simulink subsystem "AdasCorePlantModel"  (R2023a)
settings: Solver=VariableStepAuto  StartTime=0.0  StopTime=10.0  RelTol=1e-3
undefined symbols (not defined in the file or in its folder): BalNotActWait, BalOffWait, BalOnWait, Battery, contactorTime, CtrlBcuTrlrBrkGain, CtrlTcuInitGear, CtrlVcuCltch1InitCmd, CtrlVcuEvChrgLmtBpt, CtrlVcuEvRegenBrkCutOff, CtrlVcuEvRegenBrkSpdBpt, CtrlVcuEvSocBpt, currentFactor, CV_Gain, DiscIntNeverNeededParam, EnvAbsPrs, EnvAirTemp, EnvNomFrictionScaling, EnvNominalGrade, EnvWindVelX, EnvWindVelY, EnvWindVelZ, flgEnBalancing, HighTempLimit, I_cc, LowTempLimit, MaxCellVoltThrsld, MaxChrgCurrLim, MaxDchrgCurrLim, MinCellVoltDchrgCurrentLim_BP, MinCellVoltDchrgCurrentLim_Table, noCurrent, OverCellVoltageLimit, PlntBattModNumCellPar, PlntBattModNumCellSer, PlntBattNumMod, PlntBattSocInit, PlntBattTempInitDegC, PlntBrkActrBoreFrnt, PlntBrkFrntBias, PlntBrkKinFricCffFrnt, PlntBrkNumPadsFrnt, PlntBrkPadMeanRadiusFrnt, PlntBrkPrsFctr, PlntBrkRearBias, PlntDiffrntlRatio, PlntEM1EffTbl, PlntEM1Spd, PlntEM1Trq, PlntEM1TrqEff, PlntVehDstCGFrntAxl, PlntVehDstCGRearAxl, SnsrFltThld, TargetDeltaV, timeoutContactor, timeoutCurrent, Ts, UnderCellVoltageLimit, voltThreshold, vRatio
libraries: simulink x10, sharedTrackingLibrary x2, autolibutils x1
(part 1 of 4)
settings Model: Creator=sam  LastModifiedBy=sam

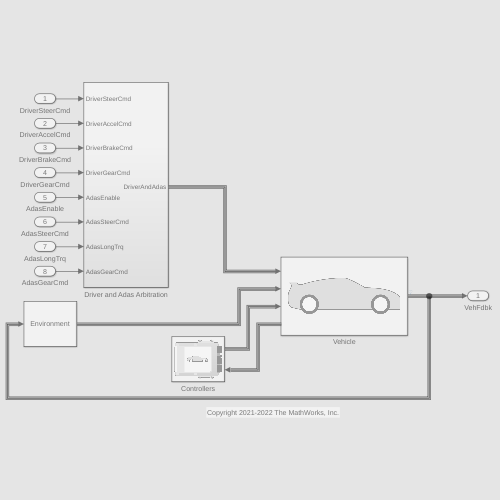
[thumbnail: Simulink's stored preview of the top-level diagram]
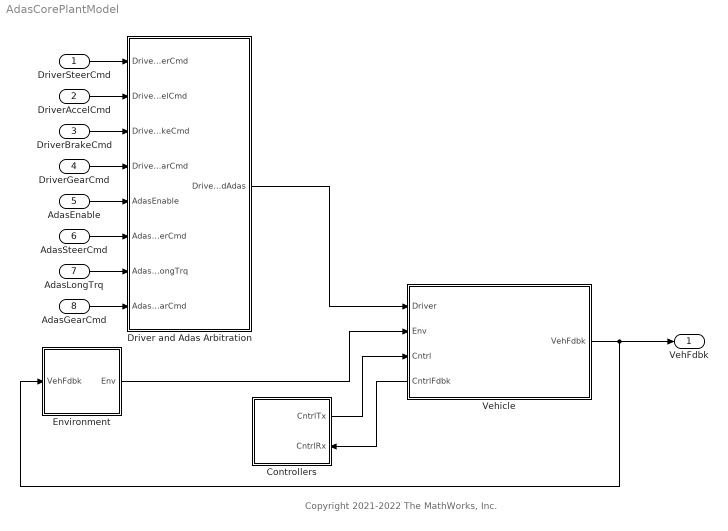
== system AdasCorePlantModel ==
  note: Copyright 2021-2022 The MathWorks, Inc.
  DriverSteerCmd : Inport
  DriverAccelCmd : Inport  Port=2
  DriverBrakeCmd : Inport  Port=3
  DriverGearCmd : Inport  Port=4
  AdasEnable : Inport  Port=5
  AdasSteerCmd : Inport  Port=6
  AdasLongTrq : Inport  Port=7
  AdasGearCmd : Inport  Port=8
  Controllers : Subsystem
      settings: PortSchema="{\"entries\":[{\"content\":{\"sides\":[{\"content\":{\"connectorIds\":[]},\"type\":\"ConnectorPlacement.EquallySpacedRectSide\",\"uuid\":\"a925dd9c-6905-4c67-a62c-b22bb69d2bd6\"},{\"content\":{\"connectorIds\":[\"Out1\",\"In1\"],\"side\":\"RIGHT\"},\"type\":\"ConnectorPlacement.EquallySpacedRectSide\",\"uuid\":\"9930ed3e-43a4-46d4-b9ee-7ed64fae32ef\"},{\"content\":{\"connectorIds\":[],\"side\":\"TOP\"},\"type\":\"ConnectorPlacement.EquallySpacedRectSide\",\"uuid\":\"68d2ac4e-de3d-40d3-8b44-059f2a72a6bc\"}]},\"type\":\"ConnectorPlacement.EquallySpacedConnector\",\"uuid\":\"c0be7d07-475b-4046-8bfa-76004f6da9b2\"}],\"packageUris\":[\"http://schema.mathworks.com/mf0/Connector/R2020b\"],\"version\":\"1.0\"}"
      mask Display: image('SystemControllers.png')
  Driver and Adas Arbitration : Subsystem
  Environment : Subsystem
      mask Display: disp('Environment')
  Vehicle : Subsystem
      settings: PortSchema="{\"entries\":[{\"content\":{\"sides\":[{\"content\":{\"connectorIds\":[\"In1\",\"In2\",\"In3\",\"Out2\"]},\"type\":\"ConnectorPlacement.EquallySpacedRectSide\",\"uuid\":\"5a3b6452-81f2-4c00-bf1f-ccfcf792e289\"},{\"content\":{\"connectorIds\":[\"Out1\"],\"side\":\"RIGHT\"},\"type\":\"ConnectorPlacement.EquallySpacedRectSide\",\"uuid\":\"1578d241-3f7e-42c3-aed7-11454fa326bd\"},{\"content\":{\"connectorIds\":[],\"side\":\"TOP\"},\"type\":\"ConnectorPlacement.EquallySpacedRectSide\",\"uuid\":\"4d307cdf-4623-4beb-9171-96c6b8eb862e\"}]},\"type\":\"ConnectorPlacement.EquallySpacedConnector\",\"uuid\":\"daa9e8ca-739b-480d-9fe9-9a76305e5c3d\"}],\"packageUris\":[\"http://schema.mathworks.com/mf0/Connector/R2020b\"],\"version\":\"1.0\"}"
      mask Display: image('PassengerVehicle.png')
  VehFdbk : Outport
  wires:
  Environment/1(Env) -> Vehicle/2(Env)
  DriverSteerCmd/1 -> Driver and Adas Arbitration/1(DriverSteerCmd)
  DriverAccelCmd/1 -> Driver and Adas Arbitration/2(DriverAccelCmd)
  Vehicle/1(VehFdbk) -> VehFdbk/1, Environment/1(VehFdbk)
  AdasGearCmd/1 -> Driver and Adas Arbitration/8(AdasGearCmd)
  Controllers/1(CntrlTx) -> Vehicle/3(Cntrl)
  DriverGearCmd/1 -> Driver and Adas Arbitration/4(DriverGearCmd)
  AdasLongTrq/1 -> Driver and Adas Arbitration/7(AdasLongTrq)
  AdasEnable/1 -> Driver and Adas Arbitration/5(AdasEnable)
  AdasSteerCmd/1 -> Driver and Adas Arbitration/6(AdasSteerCmd)
  Driver and Adas Arbitration/1(DriverAndAdas) -> Vehicle/1(Driver)
  DriverBrakeCmd/1 -> Driver and Adas Arbitration/3(DriverBrakeCmd)
  Vehicle/2(CntrlFdbk) -> Controllers/1(CntrlRx)

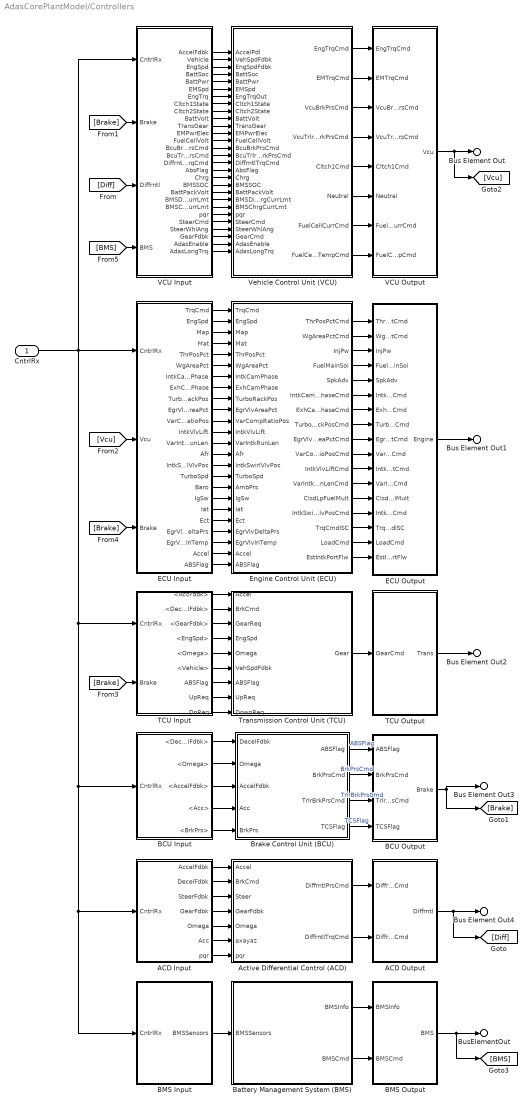
== system AdasCorePlantModel/Controllers ==
  CntrlRx : Inport
  ACD Input : Subsystem
  ACD Output : Subsystem
  Active Differential Control (ACD) : Subsystem  Variant=on  VariantControlMode=label  LabelModeActiveChoice=Choice
  BCU Input : Subsystem
  BCU Output : Subsystem
  BMS Input : Subsystem
  BMS Output : Subsystem
  Battery Management System (BMS) : Subsystem  Variant=on  VariantControlMode=label  LabelModeActiveChoice=Choice
  Brake Control Unit (BCU) : Subsystem  Variant=on  VariantControlMode=label  LabelModeActiveChoice=Choice
  ECU Input : Subsystem
  ECU Output : Subsystem
  Engine Control Unit (ECU) : Subsystem  Variant=on  VariantControlMode=label  LabelModeActiveChoice=No Engine Controller
  TCU Input : Subsystem
  TCU Output : Subsystem
  Transmission Control Unit (TCU) : Subsystem  Variant=on  VariantControlMode=label  VariantControl=Variant1  LabelModeActiveChoice=Choice
  VCU Input : Subsystem
  VCU Output : Subsystem
  Vehicle Control Unit (VCU) : Subsystem  Variant=on  VariantControlMode=label  LabelModeActiveChoice=Choice
  Bus Element Out : Outport  PortName=CntrlTx  Element=Vcu
  Bus Element Out1 : Outport  PortName=CntrlTx  Element=Engine
  Bus Element Out2 : Outport  PortName=CntrlTx  Element=Trans
  Bus Element Out3 : Outport  PortName=CntrlTx  Element=Brake
  Bus Element Out4 : Outport  PortName=CntrlTx  Element=Diff
  BusElementOut : Outport  PortName=CntrlTx  Element=BMS
  wires:
  ECU Input/1(TrqCmd) -> Engine Control Unit (ECU)/1(TrqCmd)
  CntrlRx/1 -> VCU Input/1(CntrlRx), ECU Input/1(CntrlRx), BMS Input/1(CntrlRx), ACD Input/1(CntrlRx), BCU Input/1(CntrlRx), TCU Input/1(CntrlRx)
  VCU Input/1(AccelFdbk) -> Vehicle Control Unit (VCU)/1(AccelPdl)
  VCU Input/2(Vehicle) -> Vehicle Control Unit (VCU)/2(VehSpdFdbk)
  VCU Input/3(EngSpd) -> Vehicle Control Unit (VCU)/3(EngSpdFdbk)
  VCU Input/4(BattSoc) -> Vehicle Control Unit (VCU)/4(BattSoc)
  VCU Input/5(BattPwr) -> Vehicle Control Unit (VCU)/5(BattPwr)
  VCU Input/6(EMSpd) -> Vehicle Control Unit (VCU)/6(EMSpd)
  VCU Input/7(EngTrq) -> Vehicle Control Unit (VCU)/7(EngTrqOut)
  VCU Input/8(Cltch1State) -> Vehicle Control Unit (VCU)/8(Cltch1State)
  VCU Input/9(Cltch2State) -> Vehicle Control Unit (VCU)/9(Cltch2State)
  VCU Input/10(BattVolt) -> Vehicle Control Unit (VCU)/10(BattVolt)
  VCU Input/11(TransGear) -> Vehicle Control Unit (VCU)/11(TransGear)
  VCU Input/12(EMPwrElec) -> Vehicle Control Unit (VCU)/12(EMPwrElec)
  VCU Input/13(FuelCellVolt) -> Vehicle Control Unit (VCU)/13(FuelCellVolt)
  VCU Input/18(Chrg) -> Vehicle Control Unit (VCU)/18(Chrg)
  VCU Input/17(AbsFlag) -> Vehicle Control Unit (VCU)/17(AbsFlag)
  VCU Input/16(DiffrntlTrqCmd) -> Vehicle Control Unit (VCU)/16(DiffrntlTrqCmd)
  VCU Input/14(BcuBrkPrsCmd) -> Vehicle Control Unit (VCU)/14(BcuBrkPrsCmd)
  ECU Input/2(EngSpd) -> Engine Control Unit (ECU)/2(EngSpd)
  ECU Input/3(Map) -> Engine Control Unit (ECU)/3(Map)
  ECU Input/4(Mat) -> Engine Control Unit (ECU)/4(Mat)
  ECU Input/5(ThrPosPct) -> Engine Control Unit (ECU)/5(ThrPosPct)
  ECU Input/6(WgAreaPct) -> Engine Control Unit (ECU)/6(WgAreaPct)
  ECU Input/7(IntkCamPhase) -> Engine Control Unit (ECU)/7(IntkCamPhase)
  ECU Input/8(ExhCamPhase) -> Engine Control Unit (ECU)/8(ExhCamPhase)
  ECU Input/9(TurboRackPos) -> Engine Control Unit (ECU)/9(TurboRackPos)
  ECU Input/10(EgrVlvAreaPct) -> Engine Control Unit (ECU)/10(EgrVlvAreaPct)
  ECU Input/11(VarCompRatioPos) -> Engine Control Unit (ECU)/11(VarCompRatioPos)
  ECU Input/12(IntkVlvLift) -> Engine Control Unit (ECU)/12(IntkVlvLift)
  ECU Input/13(VarIntkRunLen) -> Engine Control Unit (ECU)/13(VarIntkRunLen)
  ECU Input/14(Afr) -> Engine Control Unit (ECU)/14(Afr)
  ECU Input/15(IntkSwirlVlvPos) -> Engine Control Unit (ECU)/15(IntkSwirlVlvPos)
  ECU Input/16(TurboSpd) -> Engine Control Unit (ECU)/16(TurboSpd)
  ECU Input/17(Baro) -> Engine Control Unit (ECU)/17(AmbPrs)
  ECU Input/18(IgSw) -> Engine Control Unit (ECU)/18(IgSw)
  ECU Input/19(Iat) -> Engine Control Unit (ECU)/19(Iat)
  ECU Input/20(Ect) -> Engine Control Unit (ECU)/20(Ect)
  ECU Input/21(EgrVlvDeltaPrs) -> Engine Control Unit (ECU)/21(EgrVlvDeltaPrs)
  ECU Input/22(EgrVlvInTemp) -> Engine Control Unit (ECU)/22(EgrVlvInTemp)
  TCU Input/8(UpReq) -> Transmission Control Unit (TCU)/8(UpReq)
  TCU Input/1(<AccFdbk>) -> Transmission Control Unit (TCU)/1(Accel)
  TCU Input/2(<DecelFdbk>) -> Transmission Control Unit (TCU)/2(BrkCmd)
  TCU Input/3(<GearFdbk>) -> Transmission Control Unit (TCU)/3(GearReq)
  TCU Input/4(<EngSpd>) -> Transmission Control Unit (TCU)/4(EngSpd)
  TCU Input/5(<Omega>) -> Transmission Control Unit (TCU)/5(Omega)
  TCU Input/6(<Vehicle>) -> Transmission Control Unit (TCU)/6(VehSpdFdbk)
  TCU Input/7(ABSFlag) -> Transmission Control Unit (TCU)/7(ABSFlag)
  TCU Input/9(DnReq) -> Transmission Control Unit (TCU)/9(DownReq)
  ACD Input/1(AccelFdbk) -> Active Differential Control (ACD)/1(Accel)
  ACD Input/2(DecelFdbk) -> Active Differential Control (ACD)/2(BrkCmd)
  ACD Input/3(SteerFdbk) -> Active Differential Control (ACD)/3(Steer)
  ACD Input/4(GearFdbk) -> Active Differential Control (ACD)/4(GearFdbk)
  ACD Input/5(Omega) -> Active Differential Control (ACD)/5(Omega)
  ACD Input/6(Acc) -> Active Differential Control (ACD)/6(axayaz)
  ACD Input/7(pqr) -> Active Differential Control (ACD)/7(pqr)
  Active Differential Control (ACD)/1(DiffrntlPrsCmd) -> ACD Output/1(DiffrntlPrsCmd)
  Active Differential Control (ACD)/2(DiffrntlTrqCmd) -> ACD Output/2(DiffrntlTrqCmd)
  ACD Output/1(Diffrntl) -> [Diff], Bus Element Out4/1
  Transmission Control Unit (TCU)/1(" Gear") -> TCU Output/1(GearCmd)
  TCU Output/1(Trans) -> Bus Element Out2/1
  Vehicle Control Unit (VCU)/1(EngTrqCmd) -> VCU Output/1(EngTrqCmd)
  Vehicle Control Unit (VCU)/2(EMTrqCmd) -> VCU Output/2(EMTrqCmd)
  Vehicle Control Unit (VCU)/3(VcuBrkPrsCmd) -> VCU Output/3(VcuBrkPrsCmd)
  Vehicle Control Unit (VCU)/5(Cltch1Cmd) -> VCU Output/5(Cltch1Cmd)
  Vehicle Control Unit (VCU)/6(Neutral) -> VCU Output/6(Neutral)
  Vehicle Control Unit (VCU)/7(FuelCellCurrCmd) -> VCU Output/7(FuelCellCurrCmd)
  Vehicle Control Unit (VCU)/8(FuelCellTempCmd) -> VCU Output/8(FuelCellTempCmd)
  BCU Output/1(Brake) -> Bus Element Out3/1, [Brake]
  Engine Control Unit (ECU)/1(ThrPosPctCmd) -> ECU Output/1(ThrPosPctCmd)
  Engine Control Unit (ECU)/2(WgAreaPctCmd) -> ECU Output/2(WgAreaPctCmd)
  Engine Control Unit (ECU)/3(InjPw) -> ECU Output/3(InjPw)
  Engine Control Unit (ECU)/4(FuelMainSoi) -> ECU Output/4(FuelMainSoi)
  Engine Control Unit (ECU)/5(SpkAdv) -> ECU Output/5(SpkAdv)
  Engine Control Unit (ECU)/6(IntkCamPhaseCmd) -> ECU Output/6(IntkCamPhaseCmd)
  Engine Control Unit (ECU)/7(ExhCamPhaseCmd) -> ECU Output/7(ExhCamPhaseCmd)
  Engine Control Unit (ECU)/8(TurboRackPosCmd) -> ECU Output/8(TurboRackPosCmd)
  Engine Control Unit (ECU)/9(EgrVlvAreaPctCmd) -> ECU Output/9(EgrVlvAreaPctCmd)
  Engine Control Unit (ECU)/10(VarCompRatioPosCmd) -> ECU Output/10(VarCompRatioPosCmd)
  Engine Control Unit (ECU)/11(IntkVlvLiftCmd) -> ECU Output/11(IntkVlvLiftCmd)
  Engine Control Unit (ECU)/12(VarIntkRunLenCmd) -> ECU Output/12(VarIntkRunLenCmd)
  Engine Control Unit (ECU)/13(ClsdLpFuelMult) -> ECU Output/13(ClsdLpFuelMult)
  Engine Control Unit (ECU)/14(IntkSwirlVlvPosCmd) -> ECU Output/14(IntkSwirlVlvPosCmd)
  Engine Control Unit (ECU)/15(TrqCmdISC) -> ECU Output/15(TrqCmdISC)
  Engine Control Unit (ECU)/16(LoadCmd) -> ECU Output/16(LoadCmd)
  Engine Control Unit (ECU)/17(EstIntkPortFlw) -> ECU Output/17(EstIntkPortFlw)
  VCU Output/1(Vcu) -> Bus Element Out/1, [Vcu]
  ECU Output/1(Engine) -> Bus Element Out1/1
  [Brake] -> VCU Input/2(Brake)
  [Diff] -> VCU Input/3(Diffrntl)
  [Vcu] -> ECU Input/2(Vcu)
  [Brake] -> TCU Input/2(Brake)
  ECU Input/23(Accel) -> Engine Control Unit (ECU)/23(Accel)
  ECU Input/24(ABSFlag) -> Engine Control Unit (ECU)/24(ABSFlag)
  [Brake] -> ECU Input/3(Brake)
  Brake Control Unit (BCU)/1(ABSFlag) -> BCU Output/1(ABSFlag)  "ABSFlag"
  Brake Control Unit (BCU)/2(BrkPrsCmd) -> BCU Output/2(BrkPrsCmd)  "BrkPrsCmd"
  Brake Control Unit (BCU)/4(TCSFlag) -> BCU Output/4(TCSFlag)  "TCSFlag"
  BCU Input/1(<DecelFdbk>) -> Brake Control Unit (BCU)/1(DecelFdbk)
  BCU Input/2(<Omega>) -> Brake Control Unit (BCU)/2(Omega)
  BCU Input/5(<BrkPrs>) -> Brake Control Unit (BCU)/5(BrkPrs)
  BCU Input/4(<Acc>) -> Brake Control Unit (BCU)/4(Acc)
  BCU Input/3(<AccelFdbk>) -> Brake Control Unit (BCU)/3(AccelFdbk)
  BMS Input/1(BMSSensors) -> Battery Management System (BMS)/1(BMSSensors)
  Battery Management System (BMS)/1(BMSInfo) -> BMS Output/1(BMSInfo)
  Battery Management System (BMS)/2(BMSCmd) -> BMS Output/2(BMSCmd)
  BMS Output/1(BMS) -> [BMS], BusElementOut/1
  [BMS] -> VCU Input/4(BMS)
  VCU Input/19(BMSSOC) -> Vehicle Control Unit (VCU)/19(BMSSOC)
  VCU Input/20(BattPackVolt) -> Vehicle Control Unit (VCU)/20(BattPackVolt)
  VCU Input/21(BMSDischrgCurrLmt) -> Vehicle Control Unit (VCU)/21(BMSDischrgCurrLmt)
  VCU Input/22(BMSChrgCurrLmt) -> Vehicle Control Unit (VCU)/22(BMSChrgCurrLmt)
  Brake Control Unit (BCU)/3(TrlrBrkPrsCmd) -> BCU Output/3(TrlrBrkPrsCmd)  "TrlrBrkPrsCmd"
  Vehicle Control Unit (VCU)/4(VcuTrlrBrkPrsCmd) -> VCU Output/4(VcuTrlrBrkPrsCmd)
  VCU Input/15(BcuTrlrBrkPrsCmd) -> Vehicle Control Unit (VCU)/15(BcuTrlrBrkPrsCmd)
  VCU Input/23(pqr) -> Vehicle Control Unit (VCU)/23(pqr)
  VCU Input/24(SteerCmd) -> Vehicle Control Unit (VCU)/24(SteerCmd)
  VCU Input/25(SteerWhlAng) -> Vehicle Control Unit (VCU)/25(SteerWhlAng)
  VCU Input/26(GearFdbk) -> Vehicle Control Unit (VCU)/26(GearCmd)
  VCU Input/27(AdasEnable) -> Vehicle Control Unit (VCU)/27(AdasEnable)
  VCU Input/28(AdasLongTrq) -> Vehicle Control Unit (VCU)/28(AdasLongTrq)

== system AdasCorePlantModel/Driver and Adas Arbitration ==
  DriverSteerCmd : Inport
  DriverAccelCmd : Inport  Port=2
  DriverBrakeCmd : Inport  Port=3
  DriverGearCmd : Inport  Port=4
  AdasEnable : Inport  Port=5
  AdasSteerCmd : Inport  Port=6
  AdasLongTrq : Inport  Port=7
  AdasGearCmd : Inport  Port=8
  Bus Creator : BusCreator  Inputs=5
  Constant : Constant
  Switch : Switch  Criteria=u2 > Threshold  SaturateOnIntegerOverflow=off  InputSameDT=off
  Switch1 : Switch  Criteria=u2 > Threshold  SaturateOnIntegerOverflow=off  InputSameDT=off
  DriverAndAdas : Outport
  tag scope: AdasEnable=global, AdasGearReq=global, AdasLongTorque=global, AdasSteerCmd=global, DriverAccelPedal=global, DriverBrakePedal=global, DriverGearReq=global, DriverSteerCmd=global
  wires:
  Bus Creator/1 -> DriverAndAdas/1
  Switch1/1 -> Bus Creator/1  "SteerCmd"
  [DriverAccelPedal] -> Bus Creator/2  "AccelCmd"
  [DriverBrakePedal] -> Bus Creator/3  "DecelCmd"
  Switch/1 -> Bus Creator/4  "GearCmd"
  Constant/1 -> Bus Creator/5  "IgnSwtch"
  [AdasGearReq] -> Switch/1
  [DriverGearReq] -> Switch/3  "GearCmd"
  [AdasEnable] -> Switch/2
  [DriverSteerCmd] -> Switch1/3
  [AdasSteerCmd] -> Switch1/1
  [AdasEnable] -> Switch1/2
  DriverSteerCmd/1 -> [DriverSteerCmd]
  DriverAccelCmd/1 -> [DriverAccelPedal]
  DriverBrakeCmd/1 -> [DriverBrakePedal]
  DriverGearCmd/1 -> [DriverGearReq]
  AdasEnable/1 -> [AdasEnable]
  AdasLongTrq/1 -> [AdasLongTorque]
  AdasSteerCmd/1 -> [AdasSteerCmd]
  AdasGearCmd/1 -> [AdasGearReq]

== system AdasCorePlantModel/Environment ==
  note: The Ground Feedback variant subsystem is automatically enabled/disabled according to the 3D Engine settings found in the Reference Generator.
      | Manually overriding this variant may result in initialization errors.
  In Bus Element8 : Inport  PortName=VehFdbk  Element=Body.InertFrm
  In Bus Element9 : Inport  PortName=VehFdbk  Element=Body.InertFrm
  In Bus Element1 : Inport  PortName=VehFdbk  Element=Body.InertFrm.Cg.Disp
  BusElementIn3 : Inport  PortName=VehFdbk  Element=Wheels.Wheels.z
  BusElementIn1 : Inport  PortName=VehFdbk  Element=Wheels.Wheels.Omega
  BusElementIn : Inport  PortName=VehFdbk  Element=Suspension.SuspChassis.Whl.Ang
  Baro_Pa : Constant  Value=EnvAbsPrs  SampleTime=0
  Bus Creator : BusCreator  Inputs=3
  Bus Creator1 : BusCreator  Inputs=5
  Constant3 : Constant  Value=EnvWindVelX  SampleTime=0
  Constant4 : Constant  Value=EnvWindVelY  SampleTime=0
  Constant5 : Constant  Value=EnvWindVelZ  SampleTime=0
  Estimated Grade : Subsystem
  Ground Feedback : Subsystem  Variant=on  VariantControlMode=label  LabelModeActiveChoice=0
  Temp_degK : Constant  Value=EnvAirTemp  SampleTime=0
  Varying Friction : Subsystem  Variant=on  VariantControlMode=label  VariantControl=Choice  LabelModeActiveChoice=0
  Vector Concatenate : Concatenate  NumInputs=3
  Env : Outport  VectorParamsAs1DForOutWhenUnconnected=off
  wires:
  Constant5/1 -> Vector Concatenate/3  "Z"
  Vector Concatenate/1 -> Bus Creator1/3  "Wind"
  Constant3/1 -> Vector Concatenate/1  "X"
  Constant4/1 -> Vector Concatenate/2  "Y"
  Ground Feedback/1(Ground) -> Bus Creator1/5, Estimated Grade/1(Gnd)  "Gnd"
  Bus Creator1/1 -> Env/1
  Temp_degK/1 -> Bus Creator1/1  "Temp"
  Baro_Pa/1 -> Bus Creator1/2  "Baro"
  In Bus Element8/1 -> Varying Friction/1(In1)
  In Bus Element9/1 -> Varying Friction/2(In2)
  In Bus Element1/1 -> Varying Friction/3(Cg)
  Varying Friction/1(FricCoeffLambda) -> Ground Feedback/1(Friction)
  Estimated Grade/1(Grade) -> Bus Creator1/4  "Grade"
  BusElementIn3/1 -> Bus Creator/1  "z"
  BusElementIn1/1 -> Bus Creator/2  "Omega"
  BusElementIn/1 -> Bus Creator/3  "WhlAng"
  Bus Creator/1 -> Ground Feedback/2(WheelFdbk)  "WheelFdbk"

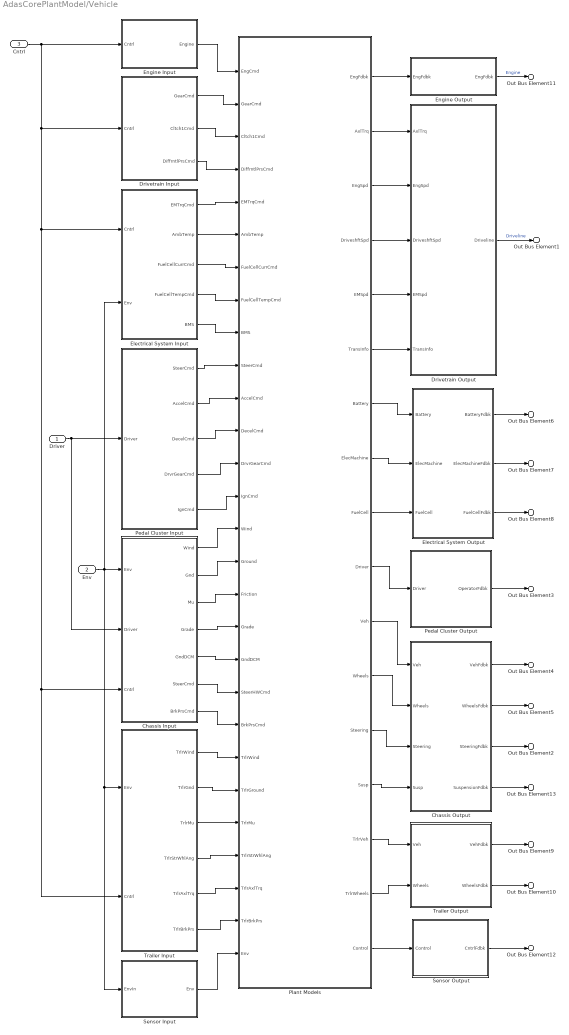
== system AdasCorePlantModel/Vehicle ==
  Driver : Inport
  Env : Inport  Port=2
  Cntrl : Inport  Port=3
  Chassis Input : Subsystem
  Chassis Output : Subsystem
  Drivetrain Input : Subsystem
  Drivetrain Output : Subsystem
  Electrical System Input : Subsystem
  Electrical System Output : Subsystem
  Engine Input : Subsystem
  Engine Output : Subsystem
  Pedal Cluster Input : Subsystem
  Pedal Cluster Output : Subsystem
  Plant Models : Subsystem  Variant=on  VariantControlMode=label  VariantControl=Choice  LabelModeActiveChoice=SimulinkModels
  Sensor Input : Subsystem
  Sensor Output : Subsystem
  Trailer Input : Subsystem
  Trailer Output : Subsystem
  Out Bus Element3 : Outport  PortName=VehFdbk  Element=Driver
  Out Bus Element4 : Outport  PortName=VehFdbk  Element=Body
  Out Bus Element5 : Outport  PortName=VehFdbk  Element=Wheels
  Out Bus Element1 : Outport  PortName=VehFdbk  Element=Driveline
  Out Bus Element2 : Outport  PortName=VehFdbk  Element=Steering
  Out Bus Element6 : Outport  PortName=VehFdbk  Element=Battery
  Out Bus Element7 : Outport  PortName=VehFdbk  Element=EM
  Out Bus Element8 : Outport  PortName=VehFdbk  Element=FuelCell
  Out Bus Element9 : Outport  PortName=VehFdbk  Element=TrlrBody
  Out Bus Element10 : Outport  PortName=VehFdbk  Element=TrlrWheels
  Out Bus Element11 : Outport  PortName=VehFdbk  Element=Engine
  Out Bus Element13 : Outport  PortName=VehFdbk  Element=Suspension
  Out Bus Element12 : Outport  Port=2  PortName=CntrlFdbk
  wires:
  Env/1 -> Electrical System Input/2(Env), Chassis Input/1(Env), Sensor Input/1(EnvIn), Trailer Input/1(Env)
  Driver/1 -> Chassis Input/2(Driver), Pedal Cluster Input/1(Driver)
  Pedal Cluster Output/1(OperatorFdbk) -> Out Bus Element3/1
  Chassis Output/2(WheelsFdbk) -> Out Bus Element5/1
  Chassis Output/1(VehFdbk) -> Out Bus Element4/1
  Drivetrain Output/1(Driveline) -> Out Bus Element1/1  "Driveline"
  Cntrl/1 -> Chassis Input/3(Cntrl), Trailer Input/2(Cntrl), Electrical System Input/1(Cntrl), Drivetrain Input/1(Cntrl), Engine Input/1(Cntrl)
  Chassis Output/3(SteeringFdbk) -> Out Bus Element2/1
  Electrical System Output/2(ElecMachineFdbk) -> Out Bus Element7/1
  Electrical System Output/1(BatteryFdbk) -> Out Bus Element6/1
  Electrical System Output/3(FuelCellFdbk) -> Out Bus Element8/1
  Trailer Output/2(WheelsFdbk) -> Out Bus Element10/1
  Trailer Output/1(VehFdbk) -> Out Bus Element9/1
  Engine Output/1(EngFdbk) -> Out Bus Element11/1  "Engine"
  Engine Input/1(Engine) -> Plant Models/1(EngCmd)
  Drivetrain Input/1(GearCmd) -> Plant Models/2(GearCmd)
  Drivetrain Input/2(Cltch1Cmd) -> Plant Models/3(Cltch1Cmd)
  Drivetrain Input/3(DiffrntlPrsCmd) -> Plant Models/4(DiffrntlPrsCmd)
  Electrical System Input/1(EMTrqCmd) -> Plant Models/5(EMTrqCmd)
  Electrical System Input/2(AmbTemp) -> Plant Models/6(AmbTemp)
  Electrical System Input/3(FuelCellCurrCmd) -> Plant Models/7(FuelCellCurrCmd)
  Electrical System Input/4(FuelCellTempCmd) -> Plant Models/8(FuelCellTempCmd)
  Pedal Cluster Input/1(SteerCmd) -> Plant Models/10(SteerCmd)
  Pedal Cluster Input/2(AccelCmd) -> Plant Models/11(AccelCmd)
  Pedal Cluster Input/3(DecelCmd) -> Plant Models/12(DecelCmd)
  Pedal Cluster Input/4(DrvrGearCmd) -> Plant Models/13(DrvrGearCmd)
  Pedal Cluster Input/5(IgnCmd) -> Plant Models/14(IgnCmd)
  Chassis Input/1(Wind) -> Plant Models/15(Wind)
  Chassis Input/2(Gnd) -> Plant Models/16(Ground)
  Chassis Input/3(Mu) -> Plant Models/17(Friction)
  Chassis Input/6(SteerCmd) -> Plant Models/20(SteerHWCmd)
  Chassis Input/7(BrkPrsCmd) -> Plant Models/21(BrkPrsCmd)
  Trailer Input/1(TrlrWind) -> Plant Models/22(TrlrWind)
  Trailer Input/2(TrlrGnd) -> Plant Models/23(TrlrGround)
  Trailer Input/3(TrlrMu) -> Plant Models/24(TrlrMu)
  Trailer Input/4(TrlrStrWhlAng) -> Plant Models/25(TrlrStrWhlAng)
  Trailer Input/5(TrlrAxlTrq) -> Plant Models/26(TrlrAxlTrq)
  Trailer Input/6(TrlrBrkPrs) -> Plant Models/27(TrlrBrkPrs)
  Plant Models/1(EngFdbk) -> Engine Output/1("EngFdbk ")
  Plant Models/2(AxlTrq) -> Drivetrain Output/1(AxlTrq)
  Plant Models/3(EngSpd) -> Drivetrain Output/2(EngSpd)
  Plant Models/4(DriveshftSpd) -> Drivetrain Output/3(DriveshftSpd)
  Plant Models/5(EMSpd) -> Drivetrain Output/4(EMSpd)
  Plant Models/6(TransInfo) -> Drivetrain Output/5(TransInfo)
  Plant Models/7(Battery) -> Electrical System Output/1(Battery)
  Plant Models/8(ElecMachine) -> Electrical System Output/2(ElecMachine)
  Plant Models/9(FuelCell) -> Electrical System Output/3(FuelCell)
  Plant Models/10(Driver) -> Pedal Cluster Output/1(Driver)
  Plant Models/11(Veh) -> Chassis Output/1(Veh)
  Plant Models/12(Wheels) -> Chassis Output/2(Wheels)
  Plant Models/13(Steering) -> Chassis Output/3(Steering)
  Plant Models/15(TrlrVeh) -> Trailer Output/1(Veh)
  Plant Models/16(TrlrWheels) -> Trailer Output/2(Wheels)
  Plant Models/17(Control) -> Sensor Output/1(Control)
  Sensor Output/1(CntrlFdbk) -> Out Bus Element12/1
  Sensor Input/1(Env) -> Plant Models/28(Env)
  Plant Models/14(Susp) -> Chassis Output/4(Susp)
  Chassis Output/4(SuspensionFdbk) -> Out Bus Element13/1
  Chassis Input/4(Grade) -> Plant Models/18(Grade)
  Electrical System Input/5(BMS) -> Plant Models/9(BMS)
  Chassis Input/5(GndDCM) -> Plant Models/19(GndDCM)

== system AdasCorePlantModel/Controllers/ACD Input ==
  CntrlRx : Inport
  Bus Selector3 : BusSelector  OutputSignals=Driver.AccelFdbk,Driver.DecelFdbk,Driver.SteerFdbk,Driver.GearFdbk,Wheels.Omega,IMU.Acc,IMU.pqr
  Rate Transition{1..7} (7 alike) : RateTransition  Deterministic=off
  AccelFdbk : Outport
  DecelFdbk : Outport  Port=2
  SteerFdbk : Outport  Port=3
  GearFdbk : Outport  Port=4
  Omega : Outport  Port=5
  Acc : Outport  Port=6
  pqr : Outport  Port=7
  wires:
  Bus Selector3/7 -> Rate Transition7/1  "<pqr>"
  Bus Selector3/3 -> Rate Transition2/1  "<SteerFdbk>"
  Bus Selector3/1 -> Rate Transition5/1  "<AccelFdbk>"
  Bus Selector3/6 -> Rate Transition6/1  "<Acc>"
  Bus Selector3/2 -> Rate Transition1/1  "<DecelFdbk>"
  Bus Selector3/4 -> Rate Transition3/1  "<GearFdbk>"
  Bus Selector3/5 -> Rate Transition4/1  "<Omega>"
  CntrlRx/1 -> Bus Selector3/1
  Rate Transition5/1 -> AccelFdbk/1
  Rate Transition1/1 -> DecelFdbk/1
  Rate Transition2/1 -> SteerFdbk/1
  Rate Transition3/1 -> GearFdbk/1
  Rate Transition4/1 -> Omega/1
  Rate Transition6/1 -> Acc/1
  Rate Transition7/1 -> pqr/1

== system AdasCorePlantModel/Controllers/ACD Output ==
  DiffrntlPrsCmd : Inport
  DiffrntlTrqCmd : Inport  Port=2
  Bus Creator4 : BusCreator  Inputs=2
  Diffrntl : Outport
  wires:
  DiffrntlPrsCmd/1 -> Bus Creator4/1  "DiffrntlPrsCmd"
  Bus Creator4/1 -> Diffrntl/1  "Diffrntl"
  DiffrntlTrqCmd/1 -> Bus Creator4/2  "DiffrntlTrqCmd"

== system AdasCorePlantModel/Controllers/Active Differential Control (ACD) ==
  note: 1) Add Subsystem or Model blocks as valid variant choices.
      | 2) You cannot connect blocks at this level. At simulation, connectivity is automatically
      | determined, based on the active variant and port name matching.
  Accel : Inport  PortDimensions=1
  BrkCmd : Inport  Port=2  PortDimensions=1
  Steer : Inport  Port=3
  GearFdbk : Inport  Port=4
  Omega : Inport  Port=5  Unit=rad/s  PortDimensions=4
  axayaz : Inport  Port=6
  pqr : Inport  Port=7
  No Control : Subsystem  VariantControl=No Control
  No Control (non-reference) : Subsystem  VariantControl=Choice
  DiffrntlPrsCmd : Outport  VectorParamsAs1DForOutWhenUnconnected=off
  DiffrntlTrqCmd : Outport  Port=2  VectorParamsAs1DForOutWhenUnconnected=off

== system AdasCorePlantModel/Controllers/BCU Input ==
  CntrlRx : Inport
  Bus Selector : BusSelector  OutputSignals=Driver.DecelFdbk,Wheels.Omega,Vehicle.xddot,Driver.AccelFdbk,Wheels.BrkPrs
  Rate Transition{1..5} (5 alike) : RateTransition  Deterministic=off
  <DecelFdbk> : Outport
  <Omega> : Outport  Port=2
  <AccelFdbk> : Outport  Port=3
  <Acc> : Outport  Port=4
  <BrkPrs> : Outport  Port=5
  wires:
  Bus Selector/4 -> Rate Transition3/1  "<AccelFdbk>"
  Bus Selector/5 -> Rate Transition4/1  "<BrkPrs>"
  Bus Selector/2 -> Rate Transition1/1  "<Omega>"
  CntrlRx/1 -> Bus Selector/1
  Bus Selector/1 -> Rate Transition5/1  "<DecelFdbk>"
  Bus Selector/3 -> Rate Transition2/1  "<xddot>"
  Rate Transition5/1 -> <DecelFdbk>/1
  Rate Transition1/1 -> <Omega>/1
  Rate Transition2/1 -> <Acc>/1
  Rate Transition3/1 -> <AccelFdbk>/1
  Rate Transition4/1 -> <BrkPrs>/1

== system AdasCorePlantModel/Controllers/BCU Output ==
  ABSFlag : Inport
  BrkPrsCmd : Inport  Port=2
  TrlrBrkPrsCmd : Inport  Port=3
  TCSFlag : Inport  Port=4
  Bus Creator2 : BusCreator  Inputs=4
  Brake : Outport
  wires:
  Bus Creator2/1 -> Brake/1  "Brake"
  BrkPrsCmd/1 -> Bus Creator2/2
  TCSFlag/1 -> Bus Creator2/4
  ABSFlag/1 -> Bus Creator2/1
  TrlrBrkPrsCmd/1 -> Bus Creator2/3

== system AdasCorePlantModel/Controllers/BMS Input ==
  CntrlRx : Inport
  Bus Selector3 : BusSelector  OutputSignals=Battery.BMSSensors
  BMSSensors : Outport
  wires:
  CntrlRx/1 -> Bus Selector3/1
  Bus Selector3/1 -> BMSSensors/1  "<BMSSensors>"

== system AdasCorePlantModel/Controllers/BMS Output ==
  BMSInfo : Inport
  BMSCmd : Inport  Port=2
  Bus Creator4 : BusCreator  Inputs=2
  BMS : Outport
  wires:
  BMSCmd/1 -> Bus Creator4/2  "BMSCmd"
  Bus Creator4/1 -> BMS/1  "BMS"
  BMSInfo/1 -> Bus Creator4/1  "BMSInfo"

== system AdasCorePlantModel/Controllers/Battery Management System (BMS) ==
  BMSSensors : Inport
  BMS (non-reference) : Subsystem  VariantControl=Choice
  Battery Management System : ModelReference  ModelNameDialog=BMSController.slx  SimulationMode=Normal  VariantControl=Battery Management System  ModelReferenceVersion=6.0
  BMSInfo : Outport
  BMSCmd : Outport  Port=2

== system AdasCorePlantModel/Controllers/Brake Control Unit (BCU) ==
  note: 1) Add Subsystem or Model blocks as valid variant choices.
      | 2) You cannot connect blocks at this level. At simulation, connectivity is automatically
      | determined, based on the active variant and port name matching.
  DecelFdbk : Inport
  Omega : Inport  Port=2
  AccelFdbk : Inport  Port=3
  Acc : Inport  Port=4
  BrkPrs : Inport  Port=5
  Open Loop Braking : ModelReference  ModelNameDialog=OpenLoopBraking  VariantControl=Open Loop  ModelReferenceVersion=2.3
  Open Loop Braking (non-reference) : Subsystem  VariantControl=Choice
  ABSFlag : Outport  VectorParamsAs1DForOutWhenUnconnected=off
  BrkPrsCmd : Outport  Port=2  VectorParamsAs1DForOutWhenUnconnected=off
  TrlrBrkPrsCmd : Outport  Port=3  VectorParamsAs1DForOutWhenUnconnected=off
  TCSFlag : Outport  Port=4  VectorParamsAs1DForOutWhenUnconnected=off

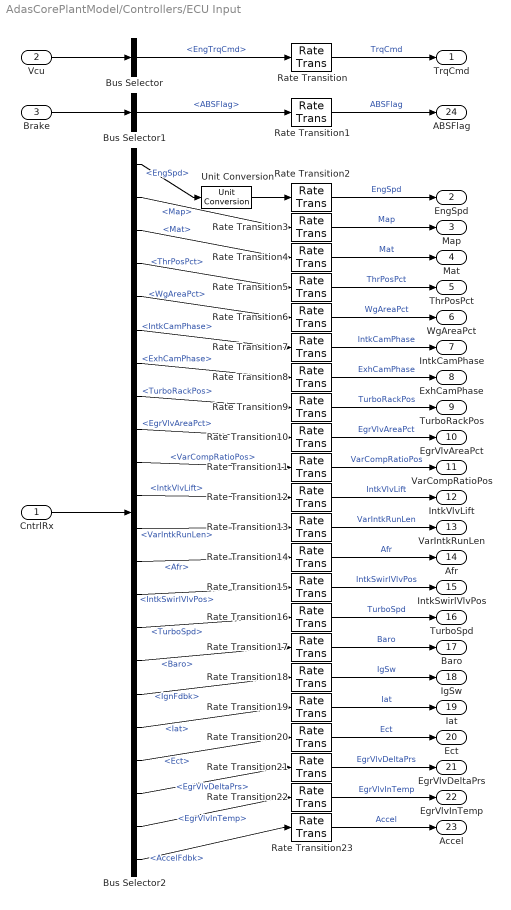
== system AdasCorePlantModel/Controllers/ECU Input ==
  CntrlRx : Inport
  Vcu : Inport  Port=2
  Brake : Inport  Port=3
  Bus Selector : BusSelector  OutputSignals=EngTrqCmd
  Bus Selector1 : BusSelector  OutputSignals=ABSFlag
  Bus Selector2 : BusSelector  OutputSignals=Trans.EngSpd,Engine.Map,Engine.Mat,Engine.ThrPosPct,Engine.WgAreaPct,Engine.IntkCamPhase,Engine.ExhCamPhase,Engine.TurboRackPos,Engine.EgrVlvAreaPct,Engine.VarCompRatioPos,Engine.IntkVlvLift,Engine.VarIntkRunLen,Engine.Afr,Engine.IntkSwirlVlvPos,Engine.TurboSpd,Env.Baro,Driver.IgnFdbk,Engine.Iat,Engine.Ect,Engine.EgrVlvDeltaPrs,Engine.EgrVlvInTemp,Driver.AccelFdbk
  Rate Transition{,1..23} (24 alike) : RateTransition  Deterministic=off
  Unit Conversion : UnitConversion
  TrqCmd : Outport
  EngSpd : Outport  Port=2
  Map : Outport  Port=3
  Mat : Outport  Port=4
  ThrPosPct : Outport  Port=5
  WgAreaPct : Outport  Port=6
  IntkCamPhase : Outport  Port=7
  ExhCamPhase : Outport  Port=8
  TurboRackPos : Outport  Port=9
  EgrVlvAreaPct : Outport  Port=10
  VarCompRatioPos : Outport  Port=11
  IntkVlvLift : Outport  Port=12
  VarIntkRunLen : Outport  Port=13
  Afr : Outport  Port=14
  IntkSwirlVlvPos : Outport  Port=15
  TurboSpd : Outport  Port=16
  Baro : Outport  Port=17
  IgSw : Outport  Port=18
  Iat : Outport  Port=19
  Ect : Outport  Port=20
  EgrVlvDeltaPrs : Outport  Port=21
  EgrVlvInTemp : Outport  Port=22
  Accel : Outport  Port=23
  ABSFlag : Outport  Port=24
  wires:
  Bus Selector2/13 -> Rate Transition14/1  "<Afr>"
  Bus Selector2/1 -> Unit Conversion/1  "<EngSpd>"
  Bus Selector2/21 -> Rate Transition22/1  "<EgrVlvInTemp>"
  Bus Selector2/19 -> Rate Transition20/1  "<Ect>"
  Bus Selector2/9 -> Rate Transition10/1  "<EgrVlvAreaPct>"
  Bus Selector2/15 -> Rate Transition16/1  "<TurboSpd>"
  Bus Selector2/17 -> Rate Transition18/1  "<IgnFdbk>"
  Bus Selector2/16 -> Rate Transition17/1  "<Baro>"
  Bus Selector2/2 -> Rate Transition3/1  "<Map>"
  Bus Selector2/18 -> Rate Transition19/1  "<Iat>"
  Bus Selector2/8 -> Rate Transition9/1  "<TurboRackPos>"
  Bus Selector2/10 -> Rate Transition11/1  "<VarCompRatioPos>"
  Bus Selector2/3 -> Rate Transition4/1  "<Mat>"
  Unit Conversion/1 -> Rate Transition2/1
  Bus Selector2/14 -> Rate Transition15/1  "<IntkSwirlVlvPos>"
  Bus Selector2/7 -> Rate Transition8/1  "<ExhCamPhase>"
  Bus Selector2/6 -> Rate Transition7/1  "<IntkCamPhase>"
  CntrlRx/1 -> Bus Selector2/1
  Bus Selector2/11 -> Rate Transition12/1  "<IntkVlvLift>"
  Bus Selector2/20 -> Rate Transition21/1  "<EgrVlvDeltaPrs>"
  Bus Selector2/12 -> Rate Transition13/1  "<VarIntkRunLen>"
  Bus Selector2/5 -> Rate Transition6/1  "<WgAreaPct>"
  Bus Selector2/4 -> Rate Transition5/1  "<ThrPosPct>"
  Bus Selector/1 -> Rate Transition/1  "<EngTrqCmd>"
  Vcu/1 -> Bus Selector/1
  Brake/1 -> Bus Selector1/1
  Bus Selector1/1 -> Rate Transition1/1  "<ABSFlag>"
  Bus Selector2/22 -> Rate Transition23/1  "<AccelFdbk>"
  Rate Transition/1 -> TrqCmd/1  "TrqCmd"
  Rate Transition1/1 -> ABSFlag/1  "ABSFlag"
  Rate Transition2/1 -> EngSpd/1  "EngSpd"
  Rate Transition3/1 -> Map/1  "Map"
  Rate Transition4/1 -> Mat/1  "Mat"
  Rate Transition5/1 -> ThrPosPct/1  "ThrPosPct"
  Rate Transition6/1 -> WgAreaPct/1  "WgAreaPct"
  Rate Transition7/1 -> IntkCamPhase/1  "IntkCamPhase"
  Rate Transition8/1 -> ExhCamPhase/1  "ExhCamPhase"
  Rate Transition9/1 -> TurboRackPos/1  "TurboRackPos"
  Rate Transition10/1 -> EgrVlvAreaPct/1  "EgrVlvAreaPct"
  Rate Transition11/1 -> VarCompRatioPos/1  "VarCompRatioPos"
  Rate Transition12/1 -> IntkVlvLift/1  "IntkVlvLift"
  Rate Transition13/1 -> VarIntkRunLen/1  "VarIntkRunLen"
  Rate Transition14/1 -> Afr/1  "Afr"
  Rate Transition15/1 -> IntkSwirlVlvPos/1  "IntkSwirlVlvPos"
  Rate Transition16/1 -> TurboSpd/1  "TurboSpd"
  Rate Transition17/1 -> Baro/1  "Baro"
  Rate Transition18/1 -> IgSw/1  "IgSw"
  Rate Transition19/1 -> Iat/1  "Iat"
  Rate Transition20/1 -> Ect/1  "Ect"
  Rate Transition21/1 -> EgrVlvDeltaPrs/1  "EgrVlvDeltaPrs"
  Rate Transition22/1 -> EgrVlvInTemp/1  "EgrVlvInTemp"
  Rate Transition23/1 -> Accel/1  "Accel"

== system AdasCorePlantModel/Controllers/ECU Output ==
  ThrPosPctCmd : Inport
  WgAreaPctCmd : Inport  Port=2
  InjPw : Inport  Port=3
  FuelMainSoi : Inport  Port=4
  SpkAdv : Inport  Port=5
  IntkCamPhaseCmd : Inport  Port=6
  ExhCamPhaseCmd : Inport  Port=7
  TurboRackPosCmd : Inport  Port=8
  EgrVlvAreaPctCmd : Inport  Port=9
  VarCompRatioPosCmd : Inport  Port=10
  IntkVlvLiftCmd : Inport  Port=11
  VarIntkRunLenCmd : Inport  Port=12
  ClsdLpFuelMult : Inport  Port=13
  IntkSwirlVlvPosCmd : Inport  Port=14
  TrqCmdISC : Inport  Port=15
  LoadCmd : Inport  Port=16
  EstIntkPortFlw : Inport  Port=17
  Bus Creator : BusCreator  Inputs=17
  Engine : Outport
  wires:
  Bus Creator/1 -> Engine/1  "Engine"
  EstIntkPortFlw/1 -> Bus Creator/17  "EstIntkPortFlw"
  ThrPosPctCmd/1 -> Bus Creator/1  "ThrPosPctCmd"
  InjPw/1 -> Bus Creator/3  "InjPw"
  SpkAdv/1 -> Bus Creator/5  "SpkAdv"
  TrqCmdISC/1 -> Bus Creator/15  "TrqCmd"
  VarCompRatioPosCmd/1 -> Bus Creator/10  "VarCompRatioPosCmd"
  FuelMainSoi/1 -> Bus Creator/4  "FuelMainSoi"
  IntkCamPhaseCmd/1 -> Bus Creator/6  "IntkCamPhaseCmd"
  ClsdLpFuelMult/1 -> Bus Creator/13  "ClsdLpFuelMult"
  WgAreaPctCmd/1 -> Bus Creator/2  "WgAreaPctCmd"
  ExhCamPhaseCmd/1 -> Bus Creator/7  "ExhCamPhaseCmd"
  TurboRackPosCmd/1 -> Bus Creator/8  "TurboRackPosCmd"
  EgrVlvAreaPctCmd/1 -> Bus Creator/9  "EgrVlvAreaPctCmd"
  IntkVlvLiftCmd/1 -> Bus Creator/11  "IntkVlvLiftCmd"
  VarIntkRunLenCmd/1 -> Bus Creator/12  "VarIntkRunLenCmd"
  IntkSwirlVlvPosCmd/1 -> Bus Creator/14  "IntkSwirlVlvPosCmd"
  LoadCmd/1 -> Bus Creator/16  "LoadCmd"

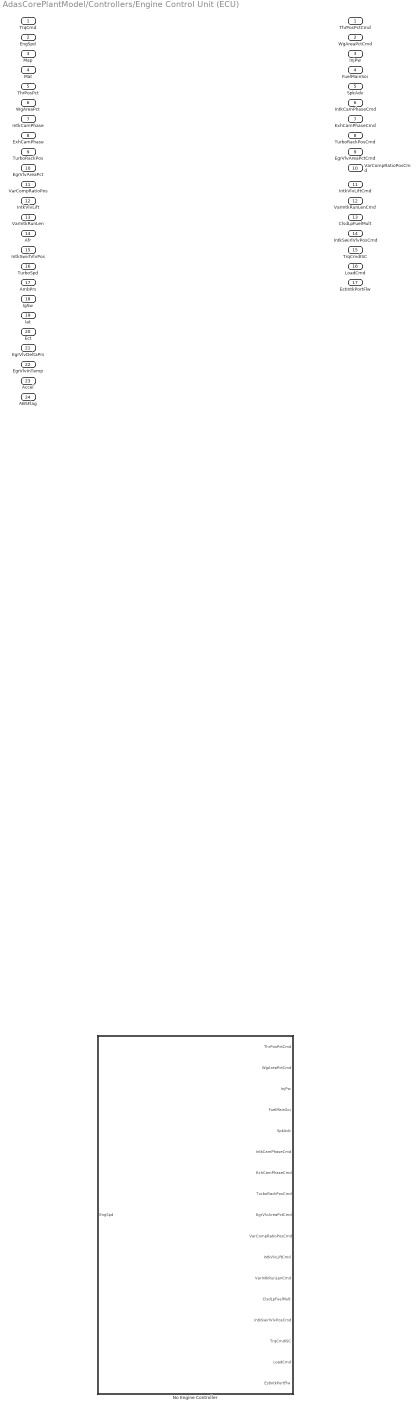
== system AdasCorePlantModel/Controllers/Engine Control Unit (ECU) ==
  TrqCmd : Inport
  EngSpd : Inport  Port=2
  Map : Inport  Port=3
  Mat : Inport  Port=4
  ThrPosPct : Inport  Port=5
  WgAreaPct : Inport  Port=6
  IntkCamPhase : Inport  Port=7
  ExhCamPhase : Inport  Port=8
  TurboRackPos : Inport  Port=9
  EgrVlvAreaPct : Inport  Port=10
  VarCompRatioPos : Inport  Port=11
  IntkVlvLift : Inport  Port=12
  VarIntkRunLen : Inport  Port=13
  Afr : Inport  Port=14
  IntkSwirlVlvPos : Inport  Port=15
  TurboSpd : Inport  Port=16
  AmbPrs : Inport  Port=17
  IgSw : Inport  Port=18
  Iat : Inport  Port=19
  Ect : Inport  Port=20
  EgrVlvDeltaPrs : Inport  Port=21
  EgrVlvInTemp : Inport  Port=22
  Accel : Inport  Port=23
  ABSFlag : Inport  Port=24
  No Engine Controller : Subsystem  VariantControl=No Engine Controller
  ThrPosPctCmd : Outport  VectorParamsAs1DForOutWhenUnconnected=off
  WgAreaPctCmd : Outport  Port=2  VectorParamsAs1DForOutWhenUnconnected=off
  InjPw : Outport  Port=3  VectorParamsAs1DForOutWhenUnconnected=off
  FuelMainSoi : Outport  Port=4  VectorParamsAs1DForOutWhenUnconnected=off
  SpkAdv : Outport  Port=5  VectorParamsAs1DForOutWhenUnconnected=off
  IntkCamPhaseCmd : Outport  Port=6  VectorParamsAs1DForOutWhenUnconnected=off
  ExhCamPhaseCmd : Outport  Port=7  VectorParamsAs1DForOutWhenUnconnected=off
  TurboRackPosCmd : Outport  Port=8  VectorParamsAs1DForOutWhenUnconnected=off
  EgrVlvAreaPctCmd : Outport  Port=9  VectorParamsAs1DForOutWhenUnconnected=off
  VarCompRatioPosCmd : Outport  Port=10  VectorParamsAs1DForOutWhenUnconnected=off
  IntkVlvLiftCmd : Outport  Port=11  VectorParamsAs1DForOutWhenUnconnected=off
  VarIntkRunLenCmd : Outport  Port=12  VectorParamsAs1DForOutWhenUnconnected=off
  ClsdLpFuelMult : Outport  Port=13  VectorParamsAs1DForOutWhenUnconnected=off
  IntkSwirlVlvPosCmd : Outport  Port=14  VectorParamsAs1DForOutWhenUnconnected=off
  TrqCmdISC : Outport  Port=15  VectorParamsAs1DForOutWhenUnconnected=off
  LoadCmd : Outport  Port=16  VectorParamsAs1DForOutWhenUnconnected=off
  EstIntkPortFlw : Outport  Port=17  VectorParamsAs1DForOutWhenUnconnected=off

== system AdasCorePlantModel/Controllers/TCU Input ==
  CntrlRx : Inport
  Brake : Inport  Port=2
  Bus Selector : BusSelector  OutputSignals=ABSFlag
  Bus Selector1 : BusSelector  OutputSignals=Driver.AccelFdbk,Driver.DecelFdbk,Driver.GearFdbk,Trans.EngSpd,Wheels.Omega,Vehicle.xdot
  Ground : Ground
  Ground1 : Ground
  Rate Transition{1..8,23} (9 alike) : RateTransition  Deterministic=off
  <AccFdbk> : Outport
  <DecelFdbk> : Outport  Port=2
  <GearFdbk> : Outport  Port=3
  <EngSpd> : Outport  Port=4
  <Omega> : Outport  Port=5
  <Vehicle> : Outport  Port=6
  ABSFlag : Outport  Port=7
  UpReq : Outport  Port=8
  DnReq : Outport  Port=9
  wires:
  Bus Selector1/6 -> Rate Transition5/1  "<xdot>"
  Bus Selector1/2 -> Rate Transition1/1  "<DecelFdbk>"
  Ground/1 -> Rate Transition7/1
  CntrlRx/1 -> Bus Selector1/1
  Bus Selector1/1 -> Rate Transition23/1  "<AccelFdbk>"
  Bus Selector1/5 -> Rate Transition4/1  "<Omega>"
  Bus Selector1/4 -> Rate Transition3/1  "<EngSpd>"
  Bus Selector1/3 -> Rate Transition2/1  "<GearFdbk>"
  Ground1/1 -> Rate Transition8/1
  Bus Selector/1 -> Rate Transition6/1  "<ABSFlag>"
  Brake/1 -> Bus Selector/1
  Rate Transition23/1 -> <AccFdbk>/1
  Rate Transition1/1 -> <DecelFdbk>/1
  Rate Transition2/1 -> <GearFdbk>/1
  Rate Transition3/1 -> <EngSpd>/1
  Rate Transition4/1 -> <Omega>/1
  Rate Transition5/1 -> <Vehicle>/1
  Rate Transition6/1 -> ABSFlag/1
  Rate Transition7/1 -> UpReq/1
  Rate Transition8/1 -> DnReq/1

== system AdasCorePlantModel/Controllers/TCU Output ==
  GearCmd : Inport
  Bus Creator1 : BusCreator  Inputs=1
  Trans : Outport
  wires:
  Bus Creator1/1 -> Trans/1  "Trans"
  GearCmd/1 -> Bus Creator1/1  "GearCmd"

== system AdasCorePlantModel/Controllers/Transmission Control Unit (TCU) ==
  Accel : Inport
  BrkCmd : Inport  Port=2
  GearReq : Inport  Port=3
  EngSpd : Inport  Port=4
  Omega : Inport  Port=5  Unit=rad/s
  VehSpdFdbk : Inport  Port=6
  ABSFlag : Inport  Port=7
  UpReq : Inport  Port=8
  DownReq : Inport  Port=9  Unit=rad/s
  DriverPassThrough : Subsystem  VariantControl=Choice
  " Gear" : Outport  VectorParamsAs1DForOutWhenUnconnected=off

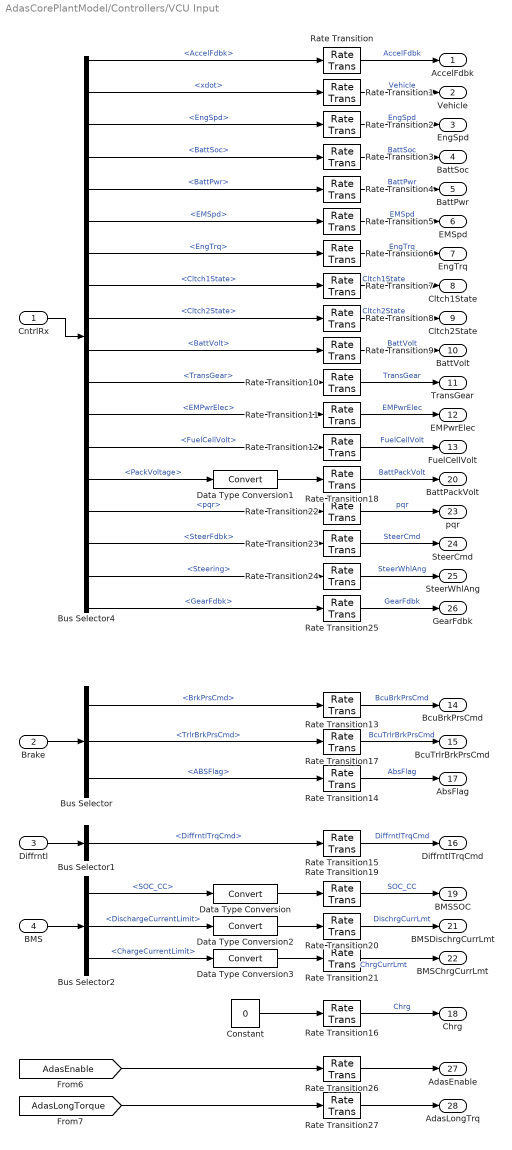
== system AdasCorePlantModel/Controllers/VCU Input ==
  CntrlRx : Inport
  Brake : Inport  Port=2
  Diffrntl : Inport  Port=3
  BMS : Inport  Port=4
  Bus Selector : BusSelector  OutputSignals=BrkPrsCmd,TrlrBrkPrsCmd,ABSFlag
  Bus Selector1 : BusSelector  OutputSignals=DiffrntlTrqCmd
  Bus Selector2 : BusSelector  OutputSignals=BMSInfo.SOC.SOC_CC,BMSCmd.CurrentLimitsBus.DischargeCurrentLimit,BMSCmd.CurrentLimitsBus.ChargeCurrentLimit
  Bus Selector4 : BusSelector  OutputSignals=Driver.AccelFdbk,Vehicle.xdot,Trans.EngSpd,Battery.BattSoc,Battery.BattPwr,Trans.EMSpd,Engine.EngTrq,Trans.Cltch1State,Trans.Cltch2State,Battery.BattVolt,Trans.TransGear,EM.EMPwrElec,FuelCell.FuelCellVolt,Battery.BMSSensors.PackVoltage,IMU.pqr,Driver.SteerFdbk,Steering,Driver.GearFdbk
  Constant : Constant  Value=0  SampleTime=-1
  Data Type Conversion{,1..3} (4 alike) : DataTypeConversion  SaturateOnIntegerOverflow=off  RndMeth=Floor
  Rate Transition{,1..27} (28 alike) : RateTransition  Deterministic=off
  AccelFdbk : Outport
  Vehicle : Outport  Port=2
  EngSpd : Outport  Port=3
  BattSoc : Outport  Port=4
  BattPwr : Outport  Port=5
  EMSpd : Outport  Port=6
  EngTrq : Outport  Port=7
  Cltch1State : Outport  Port=8
  Cltch2State : Outport  Port=9
  BattVolt : Outport  Port=10
  TransGear : Outport  Port=11
  EMPwrElec : Outport  Port=12
  FuelCellVolt : Outport  Port=13
  BcuBrkPrsCmd : Outport  Port=14
  BcuTrlrBrkPrsCmd : Outport  Port=15
  DiffrntlTrqCmd : Outport  Port=16
  AbsFlag : Outport  Port=17
  Chrg : Outport  Port=18
  BMSSOC : Outport  Port=19
  BattPackVolt : Outport  Port=20
  BMSDischrgCurrLmt : Outport  Port=21
  BMSChrgCurrLmt : Outport  Port=22
  pqr : Outport  Port=23
  SteerCmd : Outport  Port=24
  SteerWhlAng : Outport  Port=25
  GearFdbk : Outport  Port=26
  AdasEnable : Outport  Port=27
  AdasLongTrq : Outport  Port=28
  wires:
  Bus Selector4/5 -> Rate Transition4/1  "<BattPwr>"
  Bus Selector4/1 -> Rate Transition/1  "<AccelFdbk>"
  Bus Selector4/7 -> Rate Transition6/1  "<EngTrq>"
  Bus Selector4/4 -> Rate Transition3/1  "<BattSoc>"
  Bus Selector4/6 -> Rate Transition5/1  "<EMSpd>"
  CntrlRx/1 -> Bus Selector4/1
  Bus Selector4/11 -> Rate Transition10/1  "<TransGear>"
  Bus Selector4/9 -> Rate Transition8/1  "<Cltch2State>"
  Bus Selector4/13 -> Rate Transition12/1  "<FuelCellVolt>"
  Bus Selector4/8 -> Rate Transition7/1  "<Cltch1State>"
  Bus Selector4/10 -> Rate Transition9/1  "<BattVolt>"
  Bus Selector4/3 -> Rate Transition2/1  "<EngSpd>"
  Bus Selector4/12 -> Rate Transition11/1  "<EMPwrElec>"
  Bus Selector/1 -> Rate Transition13/1  "<BrkPrsCmd>"
  Constant/1 -> Rate Transition16/1
  Brake/1 -> Bus Selector/1
  Bus Selector/3 -> Rate Transition14/1  "<ABSFlag>"
  Diffrntl/1 -> Bus Selector1/1
  Bus Selector1/1 -> Rate Transition15/1  "<DiffrntlTrqCmd>"
  Rate Transition/1 -> AccelFdbk/1  "AccelFdbk"
  Rate Transition1/1 -> Vehicle/1  "Vehicle"
  Rate Transition2/1 -> EngSpd/1  "EngSpd"
  Rate Transition3/1 -> BattSoc/1  "BattSoc"
  Rate Transition4/1 -> BattPwr/1  "BattPwr"
  Rate Transition5/1 -> EMSpd/1  "EMSpd"
  Rate Transition6/1 -> EngTrq/1  "EngTrq"
  Rate Transition7/1 -> Cltch1State/1  "Cltch1State"
  Rate Transition8/1 -> Cltch2State/1  "Cltch2State"
  Rate Transition9/1 -> BattVolt/1  "BattVolt"
  Rate Transition10/1 -> TransGear/1  "TransGear"
  Rate Transition11/1 -> EMPwrElec/1  "EMPwrElec"
  Rate Transition12/1 -> FuelCellVolt/1  "FuelCellVolt"
  Rate Transition13/1 -> BcuBrkPrsCmd/1  "BcuBrkPrsCmd"
  Rate Transition14/1 -> AbsFlag/1  "AbsFlag"
  Rate Transition15/1 -> DiffrntlTrqCmd/1  "DiffrntlTrqCmd"
  Rate Transition16/1 -> Chrg/1  "Chrg"
  Rate Transition20/1 -> BMSDischrgCurrLmt/1  "DischrgCurrLmt"
  Rate Transition19/1 -> BMSSOC/1  "SOC_CC"
  Rate Transition21/1 -> BMSChrgCurrLmt/1  "ChrgCurrLmt"
  Data Type Conversion3/1 -> Rate Transition21/1
  Data Type Conversion2/1 -> Rate Transition20/1
  Bus Selector2/1 -> Data Type Conversion/1  "<SOC_CC>"
  Data Type Conversion/1 -> Rate Transition19/1
  Bus Selector2/3 -> Data Type Conversion3/1  "<ChargeCurrentLimit>"
  Bus Selector2/2 -> Data Type Conversion2/1  "<DischargeCurrentLimit>"
  BMS/1 -> Bus Selector2/1
  Data Type Conversion1/1 -> Rate Transition18/1
  Rate Transition18/1 -> BattPackVolt/1  "BattPackVolt"
  Bus Selector4/14 -> Data Type Conversion1/1  "<PackVoltage>"
  Bus Selector/2 -> Rate Transition17/1  "<TrlrBrkPrsCmd>"
  Rate Transition17/1 -> BcuTrlrBrkPrsCmd/1  "BcuTrlrBrkPrsCmd"
  Rate Transition22/1 -> pqr/1  "pqr"
  Rate Transition23/1 -> SteerCmd/1  "SteerCmd"
  Rate Transition24/1 -> SteerWhlAng/1  "SteerWhlAng"
  Bus Selector4/15 -> Rate Transition22/1  "<pqr>"
  Bus Selector4/16 -> Rate Transition23/1  "<SteerFdbk>"
  Bus Selector4/17 -> Rate Transition24/1  "<Steering>"
  Bus Selector4/2 -> Rate Transition1/1  "<xdot>"
  Rate Transition25/1 -> GearFdbk/1  "GearFdbk"
  Bus Selector4/18 -> Rate Transition25/1  "<GearFdbk>"
  [AdasEnable] -> Rate Transition26/1
  [AdasLongTorque] -> Rate Transition27/1
  Rate Transition26/1 -> AdasEnable/1
  Rate Transition27/1 -> AdasLongTrq/1

== system AdasCorePlantModel/Controllers/VCU Output ==
  EngTrqCmd : Inport
  EMTrqCmd : Inport  Port=2
  VcuBrkPrsCmd : Inport  Port=3
  VcuTrlrBrkPrsCmd : Inport  Port=4
  Cltch1Cmd : Inport  Port=5
  Neutral : Inport  Port=6
  FuelCellCurrCmd : Inport  Port=7
  FuelCellTempCmd : Inport  Port=8
  Bus Creator5 : BusCreator  Inputs=8
  Vcu : Outport
  wires:
  Cltch1Cmd/1 -> Bus Creator5/5  "Cltch1Cmd"
  EngTrqCmd/1 -> Bus Creator5/1  "EngTrqCmd"
  Bus Creator5/1 -> Vcu/1  "Vcu"
  VcuBrkPrsCmd/1 -> Bus Creator5/3  "VcuBrkPrsCmd"
  Neutral/1 -> Bus Creator5/6  "Neutral"
  FuelCellCurrCmd/1 -> Bus Creator5/7  "FuelCellCurrCmd"
  EMTrqCmd/1 -> Bus Creator5/2  "EMTrqCmd"
  FuelCellTempCmd/1 -> Bus Creator5/8  "FuelCellTempCmd"
  VcuTrlrBrkPrsCmd/1 -> Bus Creator5/4  "VcuTrlrBrkPrsCmd"

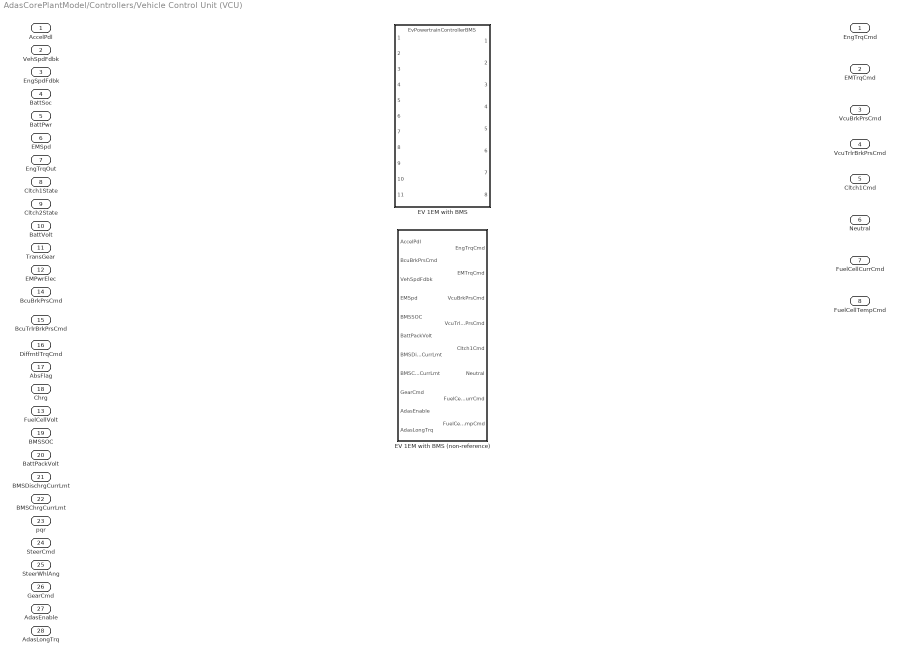
== system AdasCorePlantModel/Controllers/Vehicle Control Unit (VCU) ==
  AccelPdl : Inport
  VehSpdFdbk : Inport  Port=2
  EngSpdFdbk : Inport  Port=3
  BattSoc : Inport  Port=4
  BattPwr : Inport  Port=5
  EMSpd : Inport  Port=6
  EngTrqOut : Inport  Port=7
  Cltch1State : Inport  Port=8
  Cltch2State : Inport  Port=9
  BattVolt : Inport  Port=10
  TransGear : Inport  Port=11
  EMPwrElec : Inport  Port=12
  FuelCellVolt : Inport  Port=13
  BcuBrkPrsCmd : Inport  Port=14
  BcuTrlrBrkPrsCmd : Inport  Port=15
  DiffrntlTrqCmd : Inport  Port=16
  AbsFlag : Inport  Port=17
  Chrg : Inport  Port=18
  BMSSOC : Inport  Port=19
  BattPackVolt : Inport  Port=20
  BMSDischrgCurrLmt : Inport  Port=21
  BMSChrgCurrLmt : Inport  Port=22
  pqr : Inport  Port=23
  SteerCmd : Inport  Port=24
  SteerWhlAng : Inport  Port=25
  GearCmd : Inport  Port=26
  AdasEnable : Inport  Port=27
  AdasLongTrq : Inport  Port=28
  EV 1EM with BMS : ModelReference  ModelNameDialog=EvPowertrainControllerBMS.slx  VariantControl=EV 1EM with BMS  ModelReferenceVersion=6.37
  EV 1EM with BMS (non-reference) : Subsystem  VariantControl=Choice
  EngTrqCmd : Outport  VectorParamsAs1DForOutWhenUnconnected=off
  EMTrqCmd : Outport  Port=2  VectorParamsAs1DForOutWhenUnconnected=off
  VcuBrkPrsCmd : Outport  Port=3  VectorParamsAs1DForOutWhenUnconnected=off
  VcuTrlrBrkPrsCmd : Outport  Port=4  VectorParamsAs1DForOutWhenUnconnected=off
  Cltch1Cmd : Outport  Port=5  VectorParamsAs1DForOutWhenUnconnected=off
  Neutral : Outport  Port=6  VectorParamsAs1DForOutWhenUnconnected=off
  FuelCellCurrCmd : Outport  Port=7  VectorParamsAs1DForOutWhenUnconnected=off
  FuelCellTempCmd : Outport  Port=8  VectorParamsAs1DForOutWhenUnconnected=off

== system AdasCorePlantModel/Environment/Estimated Grade ==
  Gnd : Inport
  Atan : Trigonometry  Operator=atan
  Bus Selector : BusSelector  OutputSignals=z  OutputAsBus=on
  Bus to Vector : BusToVector
  Constant Grade : Constant  Value=EnvNominalGrade  SampleTime=-1
  Constant1 : Constant  Value=PlntVehDstCGFrntAxl+PlntVehDstCGRearAxl  SampleTime=-1
  Divide : Product  Inputs=*/
  Gain : Gain  Gain=.5
  Gain1 : Gain  Gain=.5
  Grade Source : ManualSwitch  CurrentSetting=0
  Selector : Selector  InputPortWidth=4  IndexOptions=Index vector (dialog)  Indices=[1 2]  OutputSizes=1
  Selector1 : Selector  InputPortWidth=4  IndexOptions=Index vector (dialog)  Indices=[3 4]  OutputSizes=1
  Signal Specification : SignalSpecification  Unit=rad
  Signal Specification1 : SignalSpecification  Unit=deg
  Signal Specification2 : SignalSpecification  Unit=deg
  Subtract : Sum  Inputs=+-
  Sum of Elements : Sum  Inputs=+
  Sum of Elements1 : Sum  Inputs=+
  Unit Conversion : UnitConversion
  Grade : Outport  PortDimensions=1
  wires:
  Divide/1 -> Atan/1
  Bus Selector/1 -> Bus to Vector/1
  Sum of Elements/1 -> Gain/1
  Gain/1 -> Subtract/1
  Selector/1 -> Sum of Elements/1
  Sum of Elements1/1 -> Gain1/1
  Signal Specification/1 -> Unit Conversion/1
  Constant1/1 -> Divide/2
  Selector1/1 -> Sum of Elements1/1
  Gain1/1 -> Subtract/2
  Subtract/1 -> Divide/1
  Atan/1 -> Signal Specification/1
  Grade Source/1 -> Grade/1  "Grade"
  Gnd/1 -> Bus Selector/1
  Bus to Vector/1 -> Selector1/1, Selector/1
  Constant Grade/1 -> Signal Specification2/1
  Signal Specification2/1 -> Grade Source/2
  Unit Conversion/1 -> Signal Specification1/1
  Signal Specification1/1 -> Grade Source/1  "Grade"

== system AdasCorePlantModel/Environment/Ground Feedback ==
  Friction : Inport
  WheelFdbk : Inport  Port=2
  Constant : Subsystem  VariantControl=0
  Ground : Outport  VectorParamsAs1DForOutWhenUnconnected=off

== system AdasCorePlantModel/Environment/Varying Friction ==
  In1 : Inport
  In2 : Inport  Port=2
  Cg : Inport  Port=3
  Constant Friction : Subsystem  VariantControl=0
  Varying Friction : Subsystem  VariantControl=1
  FricCoeffLambda : Outport
